simulink model "fp_sum"  (Simulink 7.6)
settings: Solver=FixedStepDiscrete  StartTime=0.0  StopTime=1  FixedStep=1  RelTol=1e-3
settings Model: Creator=jordan  LastModifiedBy=jordan
settings DataIOCC: LimitDataPoints=off  SaveOutput=off  SignalLogging=off  DSMLogging=off  SaveTime=off
settings OptimizationCC: BlockReduction=off  ConditionallyExecuteInputs=off

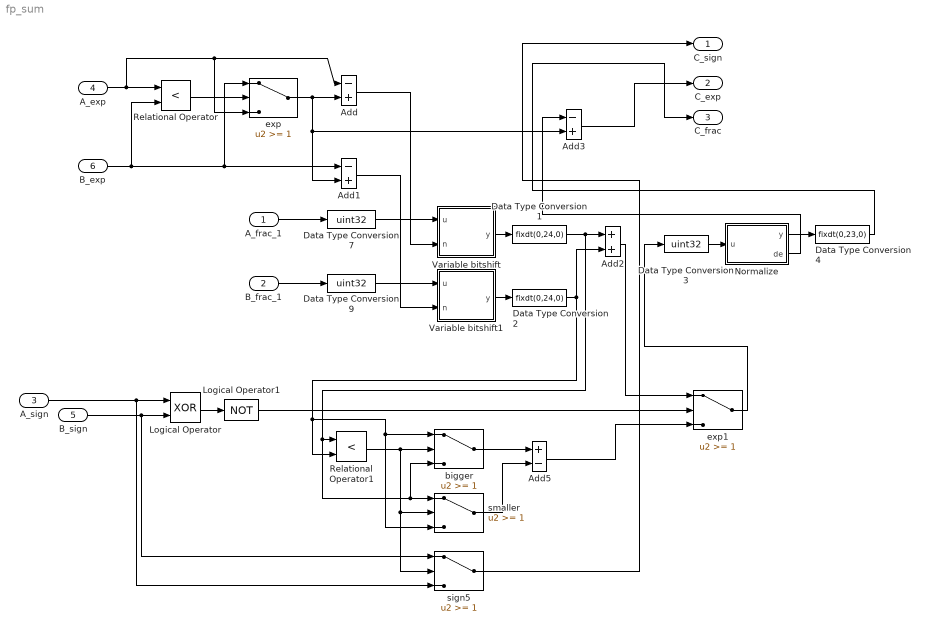
== system fp_sum ==
  A_frac_1 : Inport  OutDataTypeStr=fixdt(0,24,0)
  B_frac_1 : Inport  Port=2  OutDataTypeStr=fixdt(0,24,0)
  A_sign : Inport  Port=3  OutDataTypeStr=boolean
  A_exp : Inport  Port=4  OutDataTypeStr=uint8
  B_sign : Inport  Port=5  OutDataTypeStr=boolean
  B_exp : Inport  Port=6  OutDataTypeStr=uint8
  Add : Sum  Inputs=-+  OutDataTypeStr=int8  RndMeth=Nearest  SaturateOnIntegerOverflow=on
  Add1 : Sum  Inputs=-+  OutDataTypeStr=int8  RndMeth=Nearest  SaturateOnIntegerOverflow=on
  Add2 : Sum  OutDataTypeStr=fixdt(0,25,0)  RndMeth=Nearest  SaturateOnIntegerOverflow=on
  Add3 : Sum  Inputs=-+  OutDataTypeStr=uint8  RndMeth=Nearest  SaturateOnIntegerOverflow=on
  Add5 : Sum  Inputs=+-  OutDataTypeStr=fixdt(0,25,0)  RndMeth=Nearest  SaturateOnIntegerOverflow=on
  Data Type Conversion1 : DataTypeConversion  OutDataTypeStr=fixdt(0,24,0)
  Data Type Conversion2 : DataTypeConversion  OutDataTypeStr=fixdt(0,24,0)
  Data Type Conversion3 : DataTypeConversion  OutDataTypeStr=uint32
  Data Type Conversion4 : DataTypeConversion  OutDataTypeStr=fixdt(0,23,0)
  Data Type Conversion7 : DataTypeConversion  OutDataTypeStr=uint32
  Data Type Conversion9 : DataTypeConversion  OutDataTypeStr=uint32
  Logical Operator : Logic  Operator=XOR  AllPortsSameDT=off  OutDataTypeStr=boolean
  Logical Operator1 : Logic  Operator=NOT  AllPortsSameDT=off  OutDataTypeStr=boolean
  Normalize : Stateflow chart  TreatAsAtomicUnit=on
  Relational Operator : RelationalOperator  Operator=<  OutDataTypeStr=boolean
  Relational Operator1 : RelationalOperator  Operator=<  OutDataTypeStr=boolean
  Variable bitshift : Stateflow chart  TreatAsAtomicUnit=on
  Variable bitshift1 : Stateflow chart  TreatAsAtomicUnit=on
  bigger : Switch  Threshold=1
  exp : Switch  Threshold=1  RndMeth=Nearest
  exp1 : Switch  Threshold=1
  sign5 : Switch  Threshold=1
  smaller : Switch  Threshold=1
  C_sign : Outport  OutDataTypeStr=boolean
  C_exp : Outport  Port=2  OutDataTypeStr=uint8
  C_frac : Outport  Port=3  OutDataTypeStr=fixdt(0,23,0)
  wires:
  A_exp/1 -> Relational Operator/1, exp/3, Add/1
  B_exp/1 -> exp/1, Add1/1, Relational Operator/2
  A_frac_1/1 -> Data Type Conversion7/1
  Variable bitshift/1(y) -> Data Type Conversion1/1
  Data Type Conversion1/1 -> Add2/1, Relational Operator1/1, smaller/1, bigger/3
  Relational Operator/1 -> exp/2
  exp/1 -> Add/2, Add1/2, Add3/2
  B_frac_1/1 -> Data Type Conversion9/1
  Add/1 -> Variable bitshift/2(n)
  Add1/1 -> Variable bitshift1/2(n)
  Variable bitshift1/1(y) -> Data Type Conversion2/1
  Data Type Conversion2/1 -> Add2/2, Relational Operator1/2, bigger/1, smaller/3
  Add2/1 -> exp1/1
  Normalize/1(y) -> Data Type Conversion4/1
  Normalize/2(de) -> Add3/1
  Data Type Conversion3/1 -> Normalize/1(u)
  Data Type Conversion4/1 -> C_frac/1
  Logical Operator/1 -> Logical Operator1/1
  Logical Operator1/1 -> exp1/2
  Relational Operator1/1 -> bigger/2, smaller/2, sign5/2
  bigger/1 -> Add5/1
  smaller/1 -> Add5/2
  Add5/1 -> exp1/3
  exp1/1 -> Data Type Conversion3/1
  sign5/1 -> C_sign/1
  Data Type Conversion7/1 -> Variable bitshift/1(u)
  Data Type Conversion9/1 -> Variable bitshift1/1(u)
  A_sign/1 -> Logical Operator/1, sign5/3
  B_sign/1 -> Logical Operator/2, sign5/1
  Add3/1 -> C_exp/1

== matlab function Variable bitshift ==
  data: u input uint32; y output uint32; n input int8
function y = fcn(u,n)
%#eml

y = bitshift(u,-n);

== matlab function Variable bitshift1 ==
  data: u input uint32; y output uint32; n input int8
function y = fcn(u,n)
%#eml

y = bitshift(u,-n);

== matlab function Normalize ==
  data: u input uint32; y output uint32; de output double
function [y,de] = fcn(u)
%#eml

buf=u;
p=int8(-1);
c=bitand(buf,2^24);
for ind=1:25
    if (~c)
        p=p+1;
        buf=bitshift(buf,1);
        c=bitand(buf,2^24);
    end
end
bufy = bitand(bitshift(u,p),2^23-1);
y=bufy;
de=p;
